simulink model "RoadProfile"  (R2022a)
settings: Solver=VariableStepAuto  StartTime=0.0  StopTime=10.0  MaxStep=1e-4  RelTol=1e-3
values from neighbouring files (symbols this model uses):
  N = 500    [RandomRoadProfile.m]
  Om_max = 2*pi*10    (= 62.8318530718)    [RandomRoadProfile.m]
  Om_min = 2*pi/100    (= 0.0628318530718)    [RandomRoadProfile.m]
settings Model: Creator=s393429  LastModifiedBy=s393429

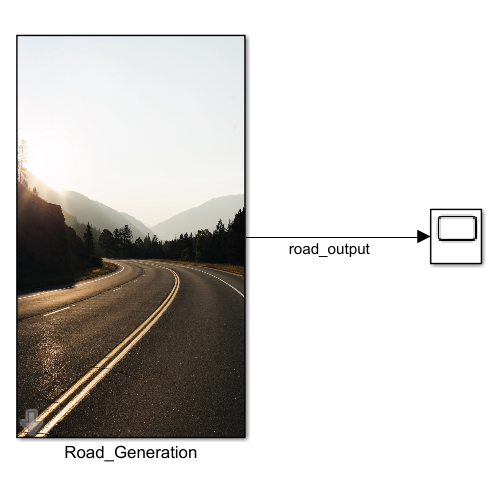
[thumbnail: Simulink's stored preview of the top-level diagram]
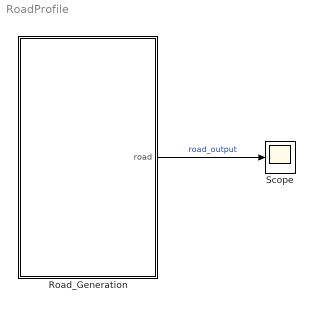
== system RoadProfile ==
  Road_Generation : Subsystem  mask{V=80, N=500, Om_min=2*pi/100, Om_max=2*pi*10, dOm=(Om_max-Om_min)/(N-1), Om_0=1, w=2, Phi_0=10e-6}
      mask prompts: V "Speed of the vehicle (km/h)"; N "Number of samples"; Om_min "Min frequency (rad/s)"; Om_max "Max frequency (rad/s)"; dOm "Space between frequency samples (rad/s)"; Om_0 "Reference Wavenumber (rad/m)"; w "Waviness"; Phi_0 "PSD at the reference wavenumber"
      mask init:
      | dOm = (Om_max-Om_min)/(N-1); % Space between frequency samples
      |     Om = Om_min:dOm:Om_max; % Frequency vector
      | 
      |     Phi = Phi_0.*(Om./Om_0).^(-w); 
      | 
      |     rng("default");
      |     Psi = 2*pi*rand(size(Om)); % Phase angles
      |     Amps = sqrt(2*Phi*dOm); % Amplitudes
      |     
      |     V = V/3.6;
      mask Display: image('road.jpg');
  Scope : Scope
  wires:
  Road_Generation/1(road) -> Scope/1  "road_output"

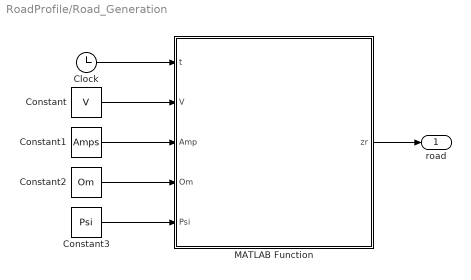
== system RoadProfile/Road_Generation ==
  Clock : Clock
  Constant : Constant  Value=V
  Constant1 : Constant  Value=Amps
  Constant2 : Constant  Value=Om
  Constant3 : Constant  Value=Psi
  MATLAB Function : MATLAB Function  TreatAsAtomicUnit=on
  road : Outport
  wires:
  Clock/1 -> MATLAB Function/1(t)
  MATLAB Function/1(zr) -> road/1
  Constant/1 -> MATLAB Function/2(V)
  Constant1/1 -> MATLAB Function/3(Amp)
  Constant2/1 -> MATLAB Function/4(Om)
  Constant3/1 -> MATLAB Function/5(Psi)

== matlab function RoadProfile/Road_Generation/MATLAB Function ==
  data: t input; zr output; V input; Amp input; Om input; Psi input
function zr = fun_02_qcm_road(t, V, Amp, Om, Psi)
% quarter car model with trailing arm suspension on random road

% pseudo random road input
s = V*t; 
u = sum(Amp.*sin(Om*s+Psi)); 
zr = u;

end
